simulink model "CoolingSpindel"  (Simulink 7.6)
settings: Solver=ode45  StartTime=0.0  StopTime=1000  RelTol=1e-3
values from neighbouring files (symbols this model uses):
  n = 0.8    [ParametersC_spindel.m]
  n1 = 0.78    [ParametersC_spindel.m]
  n2 = 0.7    [ParametersC_spindel.m]
  p = 500    [ParametersC_spindel.m]
  p1 = 380    [ParametersC_spindel.m]
  p2 = 1100    [ParametersC_spindel.m]
  R = 25    [ParametersC_spindel.m]
  sb = 5.67*(10^-8)    (= 5.67e-08)    [ParametersC_spindel.m]
  Venti_n2 = 273+40    (= 313)    [ParametersC_spindel.m]
undefined symbols (not defined in the file or in its folder): magnitude, MainDrive, MainDriveCooling
settings Model: Creator=conid  LastModifiedBy=conid

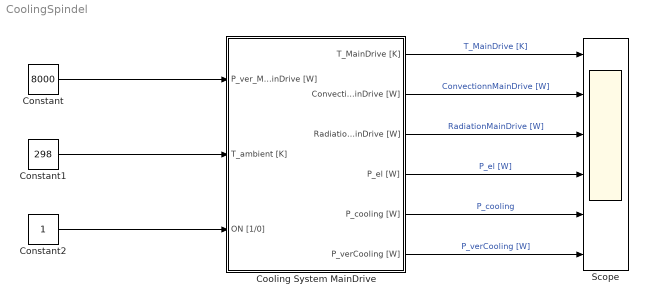
== system CoolingSpindel ==
  Constant : Constant  Value=8000
  Constant1 : Constant  Value=298
  Constant2 : Constant
  Cooling System MainDrive : Subsystem  TreatAsAtomicUnit=on
  Scope : Scope  NumInputPorts=6
      settings: YMin=-5~-5~-5~-5~-5~-5  YMax=5~5~5~5~5~5  SaveName=Scp_Cspindel
  wires:
  Constant/1 -> Cooling System MainDrive/1(P_ver_MainDrive [W])
  Constant1/1 -> Cooling System MainDrive/2(T_ambient [K])
  Constant2/1 -> Cooling System MainDrive/3(ON [1/0])
  Cooling System MainDrive/1(T_MainDrive [K]) -> Scope/1  "T_MainDrive [K]"
  Cooling System MainDrive/2(ConvectionMainDrive [W]) -> Scope/2  "ConvectionnMainDrive [W]"
  Cooling System MainDrive/3(RadiationMainDrive [W]) -> Scope/3  "RadiationMainDrive [W]"
  Cooling System MainDrive/4(P_el [W]) -> Scope/4  "P_el [W]"
  Cooling System MainDrive/5(P_cooling [W]) -> Scope/5  "P_cooling"
  Cooling System MainDrive/6(P_verCooling [W]) -> Scope/6  "P_verCooling [W]"

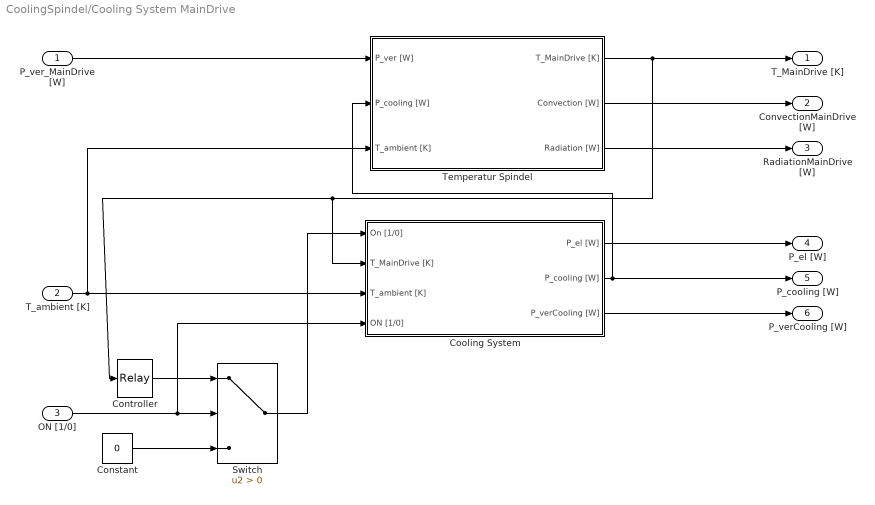
== system CoolingSpindel/Cooling System MainDrive ==
  P_ver_MainDrive [W] : Inport
  T_ambient [K] : Inport  Port=2
  ON [1/0] : Inport  Port=3
  Constant : Constant  Value=0
  Controller : Relay  OnSwitchValue=MainDriveCooling.Tmax  OffSwitchValue=MainDriveCooling.Tmin
  Cooling System : Subsystem
  Switch : Switch  Criteria=u2 > Threshold
  Temperatur Spindel : Subsystem
  T_MainDrive [K] : Outport
  ConvectionMainDrive [W] : Outport  Port=2
  RadiationMainDrive [W] : Outport  Port=3
  P_el [W] : Outport  Port=4
  P_cooling [W] : Outport  Port=5
  P_verCooling [W] : Outport  Port=6
  wires:
  P_ver_MainDrive [W]/1 -> Temperatur Spindel/1(P_ver [W])
  Constant/1 -> Switch/3
  ON [1/0]/1 -> Switch/2, Cooling System/4(ON [1/0])
  Controller/1 -> Switch/1
  Temperatur Spindel/1(T_MainDrive [K]) -> Controller/1, Cooling System/2(T_MainDrive [K]), T_MainDrive [K]/1
  Switch/1 -> Cooling System/1(On [1/0])
  T_ambient [K]/1 -> Cooling System/3(T_ambient [K]), Temperatur Spindel/3(T_ambient [K])
  Cooling System/2(P_cooling [W]) -> Temperatur Spindel/2(P_cooling [W]), P_cooling [W]/1
  Temperatur Spindel/2(Convection [W]) -> ConvectionMainDrive [W]/1
  Temperatur Spindel/3(Radiation [W]) -> RadiationMainDrive [W]/1
  Cooling System/1(P_el [W]) -> P_el [W]/1
  Cooling System/3(P_verCooling [W]) -> P_verCooling [W]/1

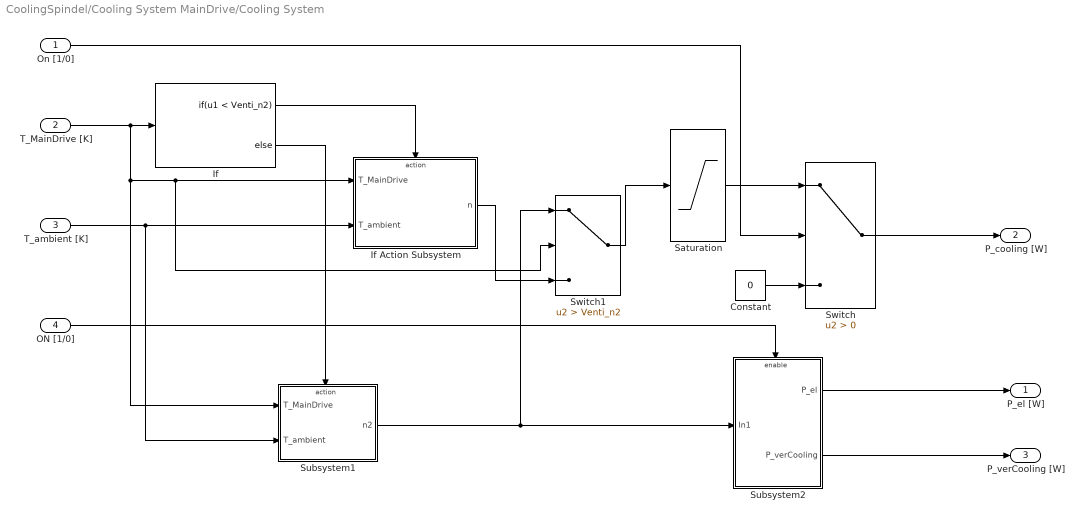
== system CoolingSpindel/Cooling System MainDrive/Cooling System ==
  On [1/0] : Inport
  T_MainDrive [K] : Inport  Port=2
  T_ambient [K] : Inport  Port=3
  ON [1/0] : Inport  Port=4
  Constant : Constant  Value=0
  If : If  IfExpression=u1 < Venti_n2
  If Action Subsystem : Subsystem  TreatAsAtomicUnit=on
  Saturation : Saturate  UpperLimit=12000  LowerLimit=0
  Subsystem1 : Subsystem
  Subsystem2 : Subsystem
  Switch : Switch  Criteria=u2 > Threshold
  Switch1 : Switch  Criteria=u2 > Threshold  Threshold=Venti_n2
  P_el [W] : Outport
  P_cooling [W] : Outport  Port=2
  P_verCooling [W] : Outport  Port=3
  wires:
  T_ambient [K]/1 -> Subsystem1/2(T_ambient), If Action Subsystem/2(T_ambient)
  Constant/1 -> Switch/3
  On [1/0]/1 -> Switch/2
  Saturation/1 -> Switch/1
  Switch/1 -> P_cooling [W]/1
  Subsystem2/1(P_el) -> P_el [W]/1
  T_MainDrive [K]/1 -> Subsystem1/1(T_MainDrive), If Action Subsystem/1(T_MainDrive), Switch1/2, If/1
  Subsystem1/1(n2) -> Switch1/1, Subsystem2/1(In1)
  ON [1/0]/1 -> Subsystem2/Enable
  Switch1/1 -> Saturation/1
  If/1 -> If Action Subsystem/Action
  If/2 -> Subsystem1/Action
  If Action Subsystem/1(n) -> Switch1/3
  Subsystem2/2(P_verCooling) -> P_verCooling [W]/1

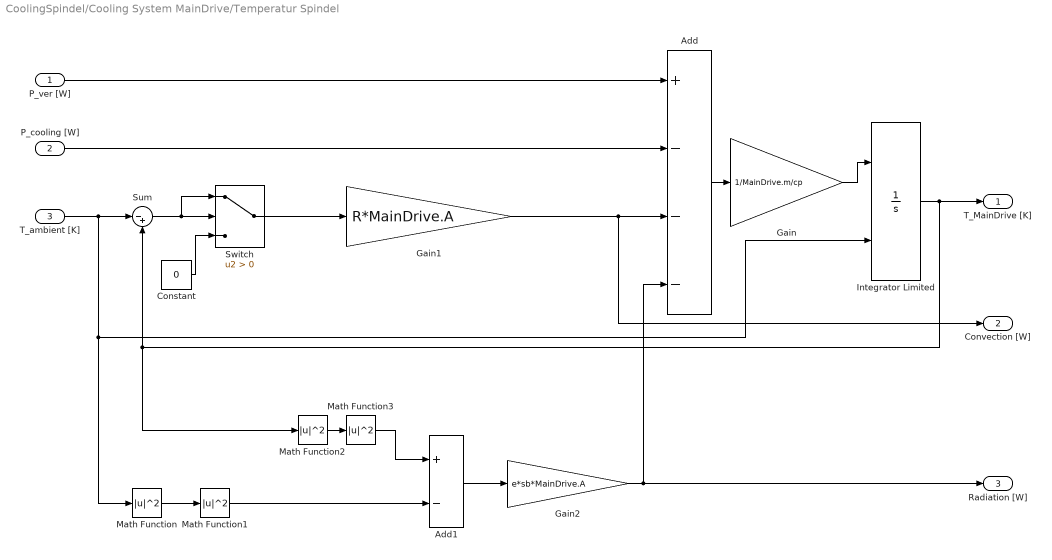
== system CoolingSpindel/Cooling System MainDrive/Temperatur Spindel ==
  P_ver [W] : Inport
  P_cooling [W] : Inport  Port=2
  T_ambient [K] : Inport  Port=3
  Add : Sum  Inputs=+---
  Add1 : Sum  Inputs=+-
  Constant : Constant  Value=0
  Gain : Gain  Gain=1/MainDrive.m/cp
  Gain1 : Gain  Gain=R*MainDrive.A
  Gain2 : Gain  Gain=e*sb*MainDrive.A
  Integrator Limited : Integrator  InitialConditionSource=external  LimitOutput=on
  Math Function{,1..3} (4 alike) : Math  Operator=magnitude^2  SaturateOnIntegerOverflow=on
  Sum : Sum  Inputs=|-+
  Switch : Switch  Criteria=u2 > Threshold
  T_MainDrive [K] : Outport
  Convection [W] : Outport  Port=2
  Radiation [W] : Outport  Port=3
  wires:
  P_ver [W]/1 -> Add/1
  Gain/1 -> Integrator Limited/1
  Gain1/1 -> Convection [W]/1, Add/3
  Integrator Limited/1 -> T_MainDrive [K]/1, Sum/2, Math Function2/1
  Add/1 -> Gain/1
  Math Function/1 -> Math Function1/1
  Gain2/1 -> Radiation [W]/1, Add/4
  P_cooling [W]/1 -> Add/2
  T_ambient [K]/1 -> Sum/1, Integrator Limited/2, Math Function/1
  Sum/1 -> Switch/2, Switch/1
  Constant/1 -> Switch/3
  Math Function2/1 -> Math Function3/1
  Add1/1 -> Gain2/1
  Math Function3/1 -> Add1/1
  Math Function1/1 -> Add1/2
  Switch/1 -> Gain1/1

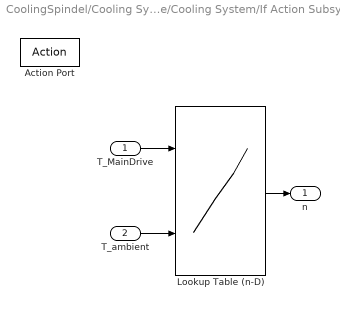
== system CoolingSpindel/Cooling System MainDrive/Cooling System/If Action Subsystem ==
  T_MainDrive : Inport
  T_ambient : Inport  Port=2
  Action Port : ActionPort  ActionType=then
  Lookup Table (n-D) : Lookup_n-D  BreakpointsForDimension1=MainDriveCooling.Air.T_int  BreakpointsForDimension2=MainDriveCooling.Air.T_ext  Table=MainDriveCooling.Air.P  InterpMethod=Cubic spline  ExtrapMethod=None - Clip  InputSameDT=on
  n : Outport
  wires:
  T_ambient/1 -> Lookup Table (n-D)/2
  T_MainDrive/1 -> Lookup Table (n-D)/1
  Lookup Table (n-D)/1 -> n/1

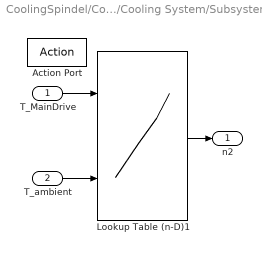
== system CoolingSpindel/Cooling System MainDrive/Cooling System/Subsystem1 ==
  T_MainDrive : Inport
  T_ambient : Inport  Port=2
  Action Port : ActionPort  ActionType=else
  Lookup Table (n-D)1 : Lookup_n-D  BreakpointsForDimension1=MainDriveCooling.Air.T_int  BreakpointsForDimension2=MainDriveCooling.Air.T_ext  Table=MainDriveCooling.Air.P_n2  InterpMethod=Cubic spline  ExtrapMethod=None - Clip  InputSameDT=on
  n2 : Outport
  wires:
  T_ambient/1 -> Lookup Table (n-D)1/2
  T_MainDrive/1 -> Lookup Table (n-D)1/1
  Lookup Table (n-D)1/1 -> n2/1

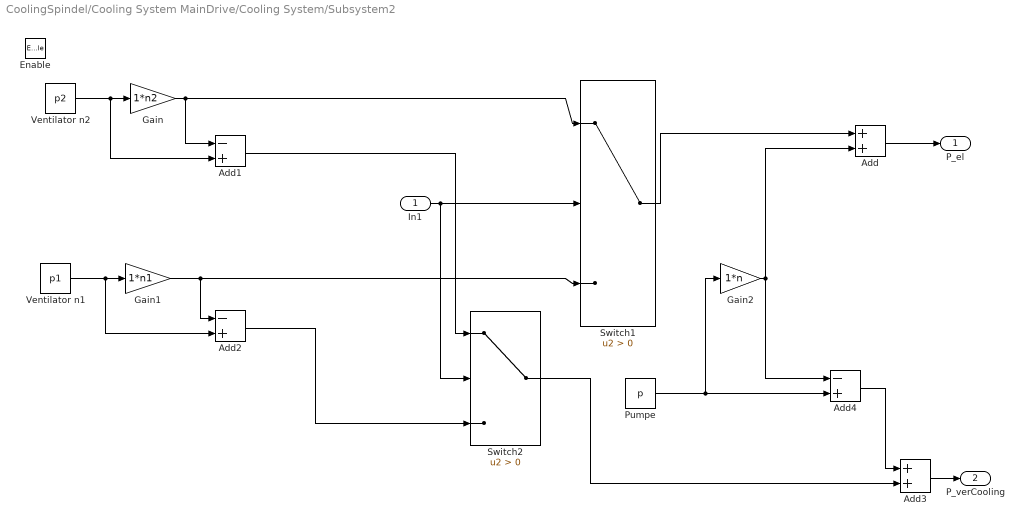
== system CoolingSpindel/Cooling System MainDrive/Cooling System/Subsystem2 ==
  In1 : Inport
  Enable : EnablePort
  Add : Sum
  Add1 : Sum  Inputs=-+
  Add2 : Sum  Inputs=-+
  Add3 : Sum
  Add4 : Sum  Inputs=-+
  Gain : Gain  Gain=1*n2
  Gain1 : Gain  Gain=1*n1
  Gain2 : Gain  Gain=1*n
  Pumpe : Constant  Value=p
  Switch1 : Switch  Criteria=u2 > Threshold
  Switch2 : Switch  Criteria=u2 > Threshold
  Ventilator n1 : Constant  Value=p1
  Ventilator n2 : Constant  Value=p2
  P_el : Outport
  P_verCooling : Outport  Port=2
  wires:
  Switch1/1 -> Add/1
  In1/1 -> Switch1/2, Switch2/2
  Add/1 -> P_el/1
  Ventilator n2/1 -> Gain/1, Add1/2
  Gain/1 -> Switch1/1, Add1/1
  Gain1/1 -> Switch1/3, Add2/1
  Ventilator n1/1 -> Gain1/1, Add2/2
  Gain2/1 -> Add/2, Add4/1
  Pumpe/1 -> Gain2/1, Add4/2
  Add4/1 -> Add3/1
  Add3/1 -> P_verCooling/1
  Add1/1 -> Switch2/1
  Add2/1 -> Switch2/3
  Switch2/1 -> Add3/2
